simulink model "pd"  (R2014b)
settings: Solver=ode45  StartTime=0.0  StopTime=10.0  RelTol=1e-3
settings Model: Creator=nlashkar  LastModifiedBy=nlashkar

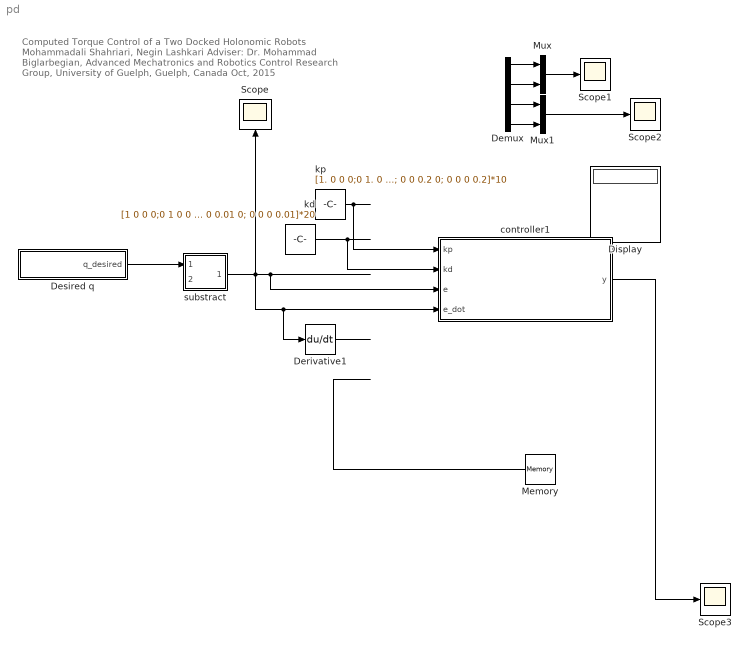
== system pd ==
  note: Computed Torque Control of a Two Docked Holonomic Robots
      | Mohammadali Shahriari, Negin Lashkari
      | Adviser: Dr. Mohammad Biglarbegian,
      | Advanced Mechatronics and Robotics Control Research Group,
      |
      | University of Guelph,
      | Guelph, Canada
      |
      | Oct, 2015
  Demux : Demux
  Derivative1 : Derivative
  "Desired q " : Subsystem
  Display : Display
  Memory : Memory  X0=[0;0;0;0;0;0;0;0]
  Mux : Mux  Inputs=2
  Mux1 : Mux  Inputs=2
  Scope{,1..3} (4 alike) : Scope
      Scope1 settings: SaveName=ScopeData2
      Scope2 settings: SaveName=ScopeData3
      Scope3 settings: SaveName=ScopeData4
  controller1 : MATLAB Function  TreatAsAtomicUnit=on
  kd : Constant  Value=[1 0 0 0;0 1 0 0 ; 0 0 0.01 0; 0 0 0 0.01]*20
  kp : Constant  Value=[1. 0 0 0;0 1. 0 0 ; 0 0 0.2 0; 0 0 0 0.2]*10
  substract : Subsystem
  wires:
  ? -> substract/2(In2)
  ? -> Display/1, Demux/1
  ? -> Memory/1
  "Desired q "/1("q_desired ") -> substract/1(In1)
  substract/1(Out1) -> controller1/3(e), controller1/4(e_dot), Derivative1/1, Scope/1
  Derivative1/1 -> ?
  kp/1 -> controller1/1(kp)
  kd/1 -> controller1/2(kd)
  Demux/1 -> Mux/1
  Demux/2 -> Mux/2
  Mux/1 -> Scope1/1
  Demux/3 -> Mux1/1
  Demux/4 -> Mux1/2
  Mux1/1 -> Scope2/1
  controller1/1(y) -> Scope3/1
  Memory/1 -> ?

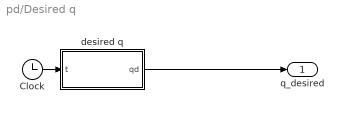
== system pd/Desired q  ==
  Clock : Clock
  desired q : MATLAB Function  TreatAsAtomicUnit=on
  "q_desired " : Outport
  wires:
  Clock/1 -> desired q/1(t)
  desired q/1(qd) -> "q_desired "/1

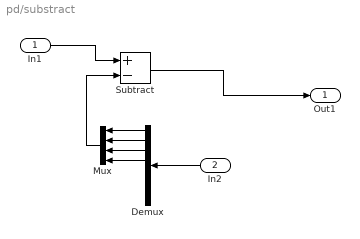
== system pd/substract ==
  In1 : Inport
  In2 : Inport  Port=2
  Demux : Demux  Outputs=8
  Mux : Mux
  Subtract : Sum  Inputs=+-
  Out1 : Outport
  wires:
  Demux/2 -> Mux/2
  Mux/1 -> Subtract/2
  Demux/1 -> Mux/1
  In1/1 -> Subtract/1
  Subtract/1 -> Out1/1
  In2/1 -> Demux/1
  Demux/3 -> Mux/3
  Demux/4 -> Mux/4

== matlab function pd/Desired q /desired q ==
  data: t input; qd output
function qd= fcn(t)
qd=q_desired(t);

== matlab function pd/controller1 ==
  data: kp input; kd input; e input; e_dot input; y output
function y= fcn(kp,kd,e,e_dot)

y=kp*e+kd*e_dot;
